simulink model "pid_testing"  (R2019b)
settings: Solver=VariableStepAuto  StartTime=0.0  StopTime=200  RelTol=1e-3
values from neighbouring files (symbols this model uses):
  B_s = 1.0e5    (= 100000)    [PID.m]
  FF_Pitch_Table = [0, 3.5, 6.0, 8.2, 10.4, 12.3, 14.0, 15.5, 18.2, 20.5, 22.5, 23.5]    [setup_model.m]
  FF_Wind_Axis = [11, 12, 13, 14, 15, 16, 17, 18, 20, 22, 24, 25]    [setup_model.m]
  J_g = 3.0e4    (= 30000)    [PID.m]
  J_r = 4.0e6    (= 4000000)    [PID.m]
  K_s = 2.0e6    (= 2000000)    [PID.m]
  Ki = (omega_n)^2 * J_r    (= 1000000)    [PID.m]
  Kp = 2 * zeta * omega_n * J_r    (= 2800000)    [PID.m]
  omega_rated = 2.0    (= 2)    [PID.m]
  R = 40    [PID.m]    (also in gen_dataset_from_sim.m)
  rho = 1.225    [PID.m]
  T_gen_max = 8.0e5    (= 800000)    [PID.m]
  T_gen_min = 0    [PID.m]
  T_gen_rated = 5.0e5    (= 500000)    [PID.m]
  tau_act = 0.05    [PID.m]
  tau_ff = 2.0    (= 2)    [setup_model.m]
libraries: simulink x4, eeGeneralControl x1
settings Model: Creator=Admin  LastModifiedBy=Admin
settings SolverCC: ZeroCrossAlgorithm=Adaptive
settings DebuggingCC: IgnoredZcDiagnostic=none

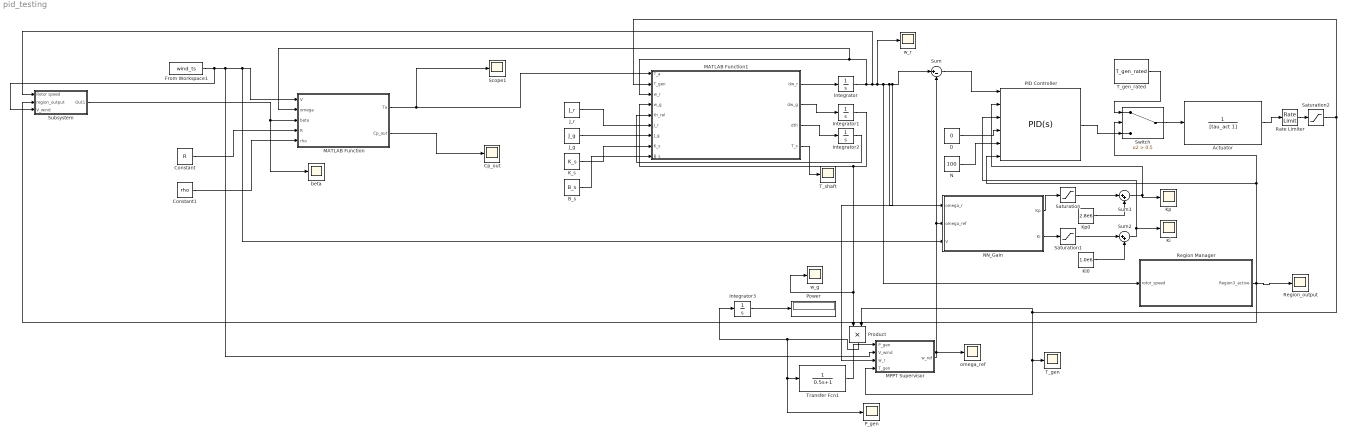
== system pid_testing ==
  Actuator : TransferFcn  Denominator=[tau_act 1]
  B_s : Constant  Value=B_s
  Constant : Constant  Value=R
  Constant1 : Constant  Value=rho
  "Cp_out " : Scope
  D : Constant  Value=0
  From Workspace1 : FromWorkspace  VariableName=wind_ts  SampleTime=0.001
  Integrator : Integrator  InitialCondition=1.5
  Integrator1 : Integrator
  Integrator2 : Integrator
  Integrator3 : Integrator
  J_g : Constant  Value=J_g
  J_r : Constant  Value=J_r
  K_s : Constant  Value=K_s
  "Ki " : Scope
  Ki0 : Constant  Value=1.0e6
  Kp : Scope
  Kp0 : Constant  Value=2.8e6
  MATLAB Function : MATLAB Function  TreatAsAtomicUnit=on
  MATLAB Function1 : MATLAB Function  TreatAsAtomicUnit=on
  "MPPT Supervisor " : Subsystem
  "N " : Constant  Value=100
  "NN_Gain " : MATLAB Function  TreatAsAtomicUnit=on
  PID Controller : simulink/Continuous/PID Controller  Controller=PID  Form=Parallel  TimeDomain=Continuous-time  SampleTime=-1  IntegratorMethod=Forward Euler  FilterMethod=Forward Euler  ControllerParametersSource=external  P=Kp  I=Ki  D=0  UseFilter=on  N=100  TunerSelectOption=Transfer Function Based (PID Tuner App)  InitialConditionSource=internal  InitialConditionForIntegrator=0  InitialConditionForFilter=0  DifferentiatorICPrevScaledInput=0  ExternalReset=level  TrackingMode=off  Kt=1  LimitOutput=on  UpperSaturationLimit=T_gen_max  LowerSaturationLimit=T_gen_min  LinearizeAsGain=on  AntiWindupMode=back-calculation  Kb=0.2  POutMin=[]  POutMax=[]  IOutMin=[]  IOutMax=[]  DOutMin=[]  DOutMax=[]  NOutMin=[]  NOutMax=[]  SumOutMin=[]  SumOutMax=[]  SaturationOutMin=[]  SaturationOutMax=[]  PParamMin=[]  PParamMax=[]  IParamMin=[]  IParamMax=[]  DParamMin=[]  DParamMax=[]  NParamMin=[]  NParamMax=[]  KbParamMin=[]  KbParamMax=[]  KtParamMin=[]  KtParamMax=[]  KbOutMin=[]  KbOutMax=[]  KtOutMin=[]  KtOutMax=[]  IntegratorOutMin=[]  IntegratorOutMax=[]  FilterOutMin=[]  FilterOutMax=[]  SumI1OutMin=[]  SumI1OutMax=[]  SumI2OutMin=[]  SumI2OutMax=[]  SumI3OutMin=[]  SumI3OutMax=[]  SumI4OutMin=[]  SumI4OutMax=[]  SumDOutMin=[]  SumDOutMax=[]  DifferentiatorOutMin=[]  DifferentiatorOutMax=[]  FilterDiffOutCoefMin=[]  FilterDiffOutCoefMax=[]  ReciprocalOutMin=[]  ReciprocalOutMax=[]  SumDenOutMin=[]  SumDenOutMax=[]  SumNumOutMin=[]  SumNumOutMax=[]  DivideOutMin=[]  DivideOutMax=[]  IntegratorContinuousStateAttributes=''  IntegratorStateMustResolveToSignalObject=off  IntegratorRTWStateStorageClass=Auto  FilterContinuousStateAttributes=''  FilterStateMustResolveToSignalObject=off  FilterRTWStateStorageClass=Auto  ParallelPVariant=ExternalParameters  IdealPVariant=Disabled  IVariant=ExternalParameters  DVariant=ExternalParameters  IntegratorVariant=Continuous  SatVariant=Enabled  AWVariant=BackCalculation  PCopyVariant=Disabled  TRVariant=Disabled  FdbkBlocksVariant=Forward  IdealPFdbkVariant=Disabled  SatFdbkVariant=Disabled  DerivativeFilterVariant=ContFilter  NVariant=ExternalParameters  NCopyVariant=Disabled  FilterICVariant=InternalICsFilter  IntegratorICVariant=InternalICs  ExternalResetVariant=ExternalReset  TRSumVariant=Passthrough  SumFdbkVariant=Disabled  SumVariant=Sum_PID
  "P_gen " : Scope
  Power : Display
  Product : Product
  Rate Limiter : RateLimiter  RisingSlewLimit=1e5  FallingSlewLimit=-1e5  SampleTimeMode=inherited
  Region Manager : Subsystem
  "Region_output " : Scope
  Saturation : Saturate  UpperLimit=8.4e5  LowerLimit=-8.4e5
  Saturation1 : Saturate  UpperLimit=3e5  LowerLimit=-3e5
  Saturation2 : Saturate  UpperLimit=8e5  LowerLimit=-8e5
  Scope1 : Scope
  Subsystem : Subsystem
  Sum : Sum  Inputs=|+-
  Sum1 : Sum  Inputs=|++
  Sum2 : Sum  Inputs=|++
  Switch : Switch  Criteria=u2 > Threshold  Threshold=0.5
  "T_gen " : Scope
  "T_gen_rated " : Constant  Value=T_gen_rated
  T_shaft : Scope
  Transfer Fcn1 : TransferFcn  Denominator=[0.5 1]
  beta : Scope
  omega_ref : Scope
  w_g : Scope
  w_r : Scope
  wires:
  MATLAB Function/1(Ta) -> Scope1/1, MATLAB Function1/1(T_a)
  Constant/1 -> MATLAB Function/4(R)
  Constant1/1 -> MATLAB Function/5(rho)
  MATLAB Function/2(Cp_out) -> "Cp_out "/1
  MATLAB Function1/3(dth) -> Integrator2/1
  MATLAB Function1/2(dw_g) -> Integrator1/1
  MATLAB Function1/1(dw_r) -> Integrator/1
  Integrator1/1 -> MATLAB Function1/4(w_g), w_g/1, Product/1
  Integrator2/1 -> MATLAB Function1/5(th_rel)
  J_r/1 -> MATLAB Function1/6(J_r)
  J_g/1 -> MATLAB Function1/7(J_g)
  K_s/1 -> MATLAB Function1/8(K_s)
  B_s/1 -> MATLAB Function1/9(B_s)
  PID Controller/1 -> Switch/3
  Sum/1 -> PID Controller/1
  D/1 -> PID Controller/4
  "N "/1 -> PID Controller/5
  "NN_Gain "/1(Kp) -> Saturation/1
  "NN_Gain "/2(Ki) -> Saturation1/1
  Saturation/1 -> Sum1/1
  Saturation1/1 -> Sum2/1
  Kp0/1 -> Sum1/2
  Ki0/1 -> Sum2/2
  Sum1/1 -> PID Controller/2, Kp/1
  Sum2/1 -> "Ki "/1, PID Controller/3
  "MPPT Supervisor "/1(w_ref) -> omega_ref/1, Sum/2, "NN_Gain "/2(omega_ref)
  Saturation2/1 -> MATLAB Function1/2(T_gen), "MPPT Supervisor "/4("T_gen "), "T_gen "/1, Product/2
  Product/1 -> "P_gen "/1, Transfer Fcn1/1, Integrator3/1
  Transfer Fcn1/1 -> "MPPT Supervisor "/1("P_gen ")
  Actuator/1 -> Rate Limiter/1
  From Workspace1/1 -> Subsystem/3("V_wind "), "MPPT Supervisor "/2("V_wind "), "NN_Gain "/3(V), MATLAB Function/1(V)
  "T_gen_rated "/1 -> Switch/1
  Switch/1 -> Actuator/1
  Subsystem/1(Out1) -> MATLAB Function/3(beta), beta/1
  Integrator3/1 -> Power/1
  Rate Limiter/1 -> Saturation2/1
  MATLAB Function1/4(T_s) -> T_shaft/1
  Region Manager/1("Region3_active ") -> Subsystem/2(region_output), "Region_output "/1, PID Controller/6, Switch/2
  Integrator/1 -> Subsystem/1(Rotor speed), Region Manager/1("rotor_speed "), "MPPT Supervisor "/3(w_r), Sum/1, "NN_Gain "/1(omega_r), w_r/1, MATLAB Function/2(omega), MATLAB Function1/3(w_r)

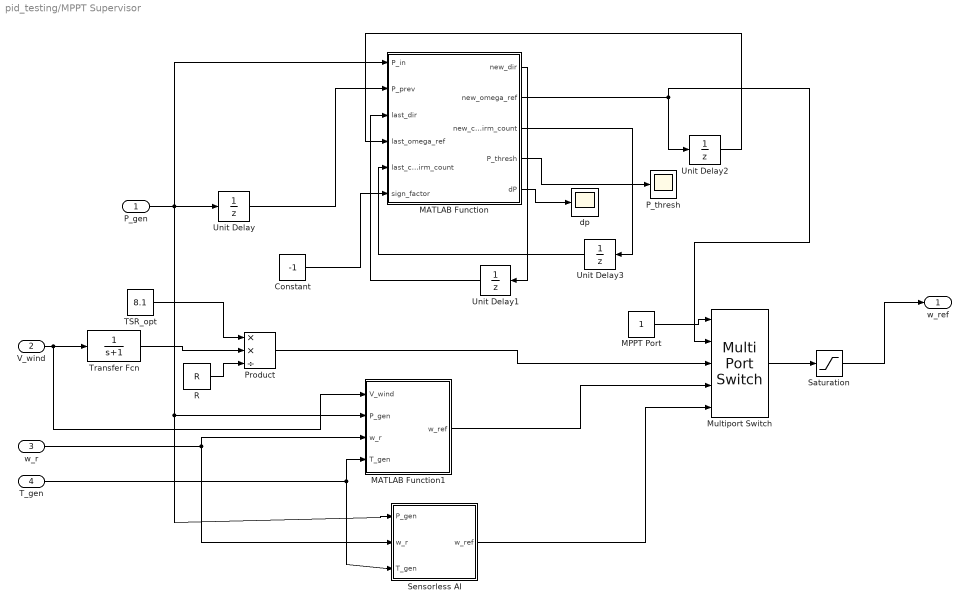
== system pid_testing/MPPT Supervisor  ==
  "P_gen " : Inport
  "V_wind " : Inport  Port=2
  w_r : Inport  Port=3
  "T_gen " : Inport  Port=4
  Constant : Constant  Value=-1
  MATLAB Function : MATLAB Function  TreatAsAtomicUnit=on
  MATLAB Function1 : MATLAB Function  TreatAsAtomicUnit=on
  MPPT Port : Constant
  Multiport Switch : MultiPortSwitch  Inputs=4
  P_thresh : Scope
  Product : Product  Inputs=**/
  "R " : Constant  Value=R
  Saturation : Saturate  UpperLimit=2.2  LowerLimit=0.7
  "Sensorless AI " : MATLAB Function  TreatAsAtomicUnit=on
  "TSR_opt " : Constant  Value=8.1
  Transfer Fcn : TransferFcn  Denominator=[1 1]
  Unit Delay : UnitDelay  HasFrameUpgradeWarning=on
  Unit Delay1 : UnitDelay  InitialCondition=1  HasFrameUpgradeWarning=on
  Unit Delay2 : UnitDelay  InitialCondition=1.5  HasFrameUpgradeWarning=on
  Unit Delay3 : UnitDelay  HasFrameUpgradeWarning=on
  "dp " : Scope
  w_ref : Outport
  wires:
  "P_gen "/1 -> "Sensorless AI "/1(P_gen), MATLAB Function1/2(P_gen), MATLAB Function/1(P_in), Unit Delay/1
  MATLAB Function/1(new_dir) -> Unit Delay1/1
  Unit Delay/1 -> MATLAB Function/2(P_prev)
  Unit Delay1/1 -> MATLAB Function/3(last_dir)
  Unit Delay2/1 -> MATLAB Function/4(last_omega_ref)
  Unit Delay3/1 -> MATLAB Function/5(last_confirm_count)
  Constant/1 -> MATLAB Function/6(sign_factor)
  MATLAB Function/2(new_omega_ref) -> Multiport Switch/2, Unit Delay2/1
  MATLAB Function/3(new_confirm_count) -> Unit Delay3/1
  MATLAB Function/4(P_thresh) -> P_thresh/1
  MATLAB Function/5(dP) -> "dp "/1
  "R "/1 -> Product/3
  "V_wind "/1 -> MATLAB Function1/1(V_wind), Transfer Fcn/1
  "TSR_opt "/1 -> Product/1
  Transfer Fcn/1 -> Product/2
  Product/1 -> Multiport Switch/3
  Multiport Switch/1 -> Saturation/1
  MPPT Port/1 -> Multiport Switch/1
  Saturation/1 -> w_ref/1
  w_r/1 -> MATLAB Function1/3(w_r), "Sensorless AI "/2(w_r)
  "T_gen "/1 -> MATLAB Function1/4(T_gen), "Sensorless AI "/3(T_gen)
  MATLAB Function1/1(w_ref) -> Multiport Switch/4
  "Sensorless AI "/1(w_ref) -> Multiport Switch/5

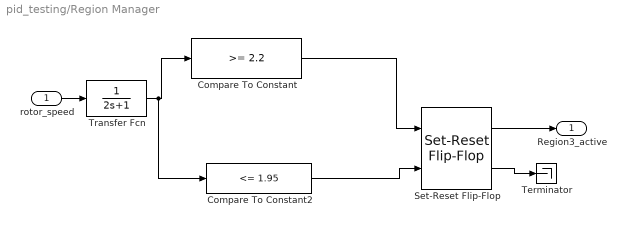
== system pid_testing/Region Manager ==
  "rotor_speed " : Inport
  Compare To Constant : simulink/Logic and Bit Operations/Compare To Constant  relop=>=  const=2.2  OutDataTypeStr=boolean
  Compare To Constant2 : simulink/Logic and Bit Operations/Compare To Constant  relop=<=  const=1.95  OutDataTypeStr=boolean
  Set-Reset Flip-Flop : eeGeneralControl/Set-Reset Flip-Flop  LabelModeActiveChoice=Discrete  UndefState=Set  Q0=0  Ts=-1
      settings: SourceProductName=Simscape Electrical  SourceProductBaseCode=PS
  Terminator : Terminator
  Transfer Fcn : TransferFcn  Denominator=[2 1]
  "Region3_active " : Outport
  wires:
  "rotor_speed "/1 -> Transfer Fcn/1
  Compare To Constant/1 -> Set-Reset Flip-Flop/1
  Compare To Constant2/1 -> Set-Reset Flip-Flop/2
  Set-Reset Flip-Flop/1 -> "Region3_active "/1
  Set-Reset Flip-Flop/2 -> Terminator/1
  Transfer Fcn/1 -> Compare To Constant2/1, Compare To Constant/1

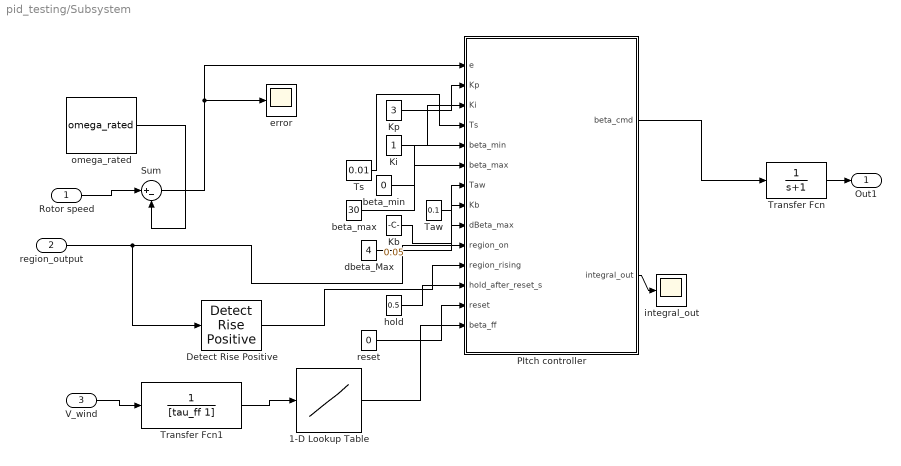
== system pid_testing/Subsystem ==
  Rotor speed : Inport
  region_output : Inport  Port=2
  "V_wind " : Inport  Port=3
  1-D Lookup Table : Lookup_n-D  NumberOfTableDimensions=1  BreakpointsForDimension1=FF_Wind_Axis  Table=FF_Pitch_Table  InternalRulePriority=Speed  RndMeth=Simplest  InputSameDT=on
  Detect Rise Positive : simulink/Logic and Bit Operations/Detect Rise Positive  vinit=0  OutDataTypeStr=boolean
  Kb : Constant  Value=0.05
  Ki : Constant
  Kp : Constant  Value=3
  "PItch controller " : MATLAB Function  TreatAsAtomicUnit=on
  Sum : Sum  Inputs=|+-
  Taw : Constant  Value=0.1
  Transfer Fcn : TransferFcn  Denominator=[1 1]
  Transfer Fcn1 : TransferFcn  Denominator=[tau_ff 1]
  Ts : Constant  Value=0.01
  beta_max : Constant  Value=30
  beta_min : Constant  Value=0
  dbeta_Max : Constant  Value=4
  error : Scope
  hold : Constant  Value=0.5
  "integral_out " : Scope
  "omega_rated " : Constant  Value=omega_rated
  reset : Constant  Value=0
  Out1 : Outport
  wires:
  Rotor speed/1 -> Sum/1
  "omega_rated "/1 -> Sum/2
  Transfer Fcn/1 -> Out1/1
  Sum/1 -> error/1, "PItch controller "/1(e)
  region_output/1 -> Detect Rise Positive/1, "PItch controller "/10(region_on)
  Kp/1 -> "PItch controller "/2(Kp)
  Ki/1 -> "PItch controller "/3(Ki)
  Ts/1 -> "PItch controller "/4(Ts)
  beta_min/1 -> "PItch controller "/5(beta_min)
  beta_max/1 -> "PItch controller "/6(beta_max)
  Taw/1 -> "PItch controller "/7(Taw)
  Kb/1 -> "PItch controller "/8(Kb)
  dbeta_Max/1 -> "PItch controller "/9(dBeta_max)
  hold/1 -> "PItch controller "/12(hold_after_reset_s)
  reset/1 -> "PItch controller "/13(reset)
  "PItch controller "/1(beta_cmd) -> Transfer Fcn/1
  "PItch controller "/2(integral_out) -> "integral_out "/1
  Detect Rise Positive/1 -> "PItch controller "/11(region_rising)
  "V_wind "/1 -> Transfer Fcn1/1
  Transfer Fcn1/1 -> 1-D Lookup Table/1
  1-D Lookup Table/1 -> "PItch controller "/14(beta_ff)

== matlab function pid_testing/MATLAB Function1 ==
  data: T_a input; dw_r output; dw_g output; dth output; T_gen input; w_r input; w_g input; th_rel input; J_r input; J_g input; K_s input; B_s input; T_s output
function [dw_r, dw_g, dth,T_s] = two_mass_dynamics_derivatives(T_a, T_gen, w_r, w_g, th_rel, J_r, J_g, K_s, B_s)
    % This function now calculates DERIVATIVES, not states.

    % Parameters (can be passed in or defined here)


    % Shaft torque calculation (based on current states)
    T_s = K_s * th_rel + B_s * (w_r - w_g);

    % Output the derivatives
    dw_r = (T_a - T_s) / J_r;
    dw_g = (T_s - T_gen) / J_g;
    dth  = w_r - w_g;
end

== matlab function pid_testing/MATLAB Function ==
  data: V input; Ta output; omega input; beta input; R input; Cp_out output; rho input
function [Ta, Cp_out] = aero_torque(V, omega, beta, R, rho)
%#codegen
% Aero torque using analytic Cp; no structs/buses required.
% Inputs:
%   V     - wind speed [m/s]
%   omega - rotor speed [rad/s]
%   beta  - pitch [deg]
%   R     - rotor radius [m]
%   rho   - air density [kg/m^3]
% Outputs:
%   Ta    - aerodynamic torque [N*m]
%   Cp_out- power coefficient (dimensionless)

% Protect inputs
if V <= 1e-6
    V = 1e-6;
end
if omega <= 1e-6
    omega = 1e-6;
end
if R <= 0
    R = 40; % fallback
end
if rho <= 0
    rho = 1.225;
end

% Tip-speed ratio
lambda = omega .* R ./ V;

% Analytic Cp coefficients (replace later with your own if needed)
c1 = 0.5176; c2 = 116; c3 = 0.4; c4 = 5; c5 = 21; c6 = 0;
% Compute lambda_i safely (avoid divide by zero)
den = 1./(lambda + 0.08.*beta) - 0.035./(beta.^3 + 1);
den(den==0) = eps;
lambda_i = 1 ./ den;

Cp_out = c1 .* ((c2 ./ lambda_i - c3 .* beta - c4) .* exp(-c5 ./ lambda_i)) + c6 .* lambda;
% enforce physical bounds
Cp_out = max(0, min(Cp_out, 0.59));

% Rotor swept area
A = pi .* R.^2;

% Aerodynamic torque (use omega-safe)
Ta = 0.5 .* rho .* A .* V.^3 .* Cp_out ./ omega;

% If V is essentially zero, set torque to zero
Ta(V < 1e-6) = 0;
end

== matlab function pid_testing/NN_Gain  ==
  settings: updateMethod=DISCRETE  sampleTime=0.1
  data: omega_r input; Kp output; omega_ref input; V input; Ki output
function [Kp, Ki] = NN_GainScheduler(omega_r, omega_ref, V)
%#codegen
% This block calls an external helper function to run the network.

% Tell the Coder that 'runMyNet' is an external MATLAB function
coder.extrinsic('runMyNet');

% --- Pre-allocate all variables for the Coder ---
% This prevents any "undefined variable" errors.
Kp = 0.0;
Ki = 0.0;
K  = zeros(2,1); % K is a 2x1 vector of doubles

% --- Format the inputs ---
x = [omega_r; omega_ref; V];

% --- Call the helper function ---
% This passes the inputs to 'runMyNet' and gets the 2x1 'K' vector back.
% All complex network logic is hidden from the Coder.
K = runMyNet(x);

% --- Assign the outputs ---
Kp = K(1);
Ki = K(2);

== matlab function pid_testing/MPPT Supervisor /MATLAB Function ==
  data: P_in input; new_dir output; P_prev input; last_dir input; last_omega_ref input; last_confirm_count input; sign_factor input; new_omega_ref output; new_confirm_count output; P_thresh output; dP output
function [new_dir, new_omega_ref, new_confirm_count, P_thresh, dP] = po_fcn( ...
    P_in, P_prev, last_dir, last_omega_ref, last_confirm_count, sign_factor)
% P&O robust step decision
% Inputs:
%  P_in   - filtered power at current step
%  P_prev - filtered power at previous step (UnitDelay)
%  last_dir - previous perturbation direction (+1 or -1) (UnitDelay)
%  last_omega_ref - previous omega_ref (UnitDelay)
%  last_confirm_count - previous consecutive-sign count (UnitDelay)
%  sign_factor - +1 or -1 to flip ΔP interpretation quickly (tune)
%
% Outputs:
%  new_dir - new perturbation direction (+1 or -1)
%  new_omega_ref - updated omega_ref (already saturated here)
%  new_confirm_count - updated confirmation counter
%  P_thresh - computed deadband threshold
%  dP - change in power (for debug/plot)

%% Parameters (tune these)
base_step = 0.02;        % rad/s base step size
min_step  = 0.01;        % minimum step size
omega_min = 0.7;         % lower bound for omega_ref
omega_max = 2.2;         % upper bound for omega_ref
P_thresh_abs = 100;      % absolute deadband [W]
P_rel_factor = 0.002;    % relative deadband fraction of P_in
confirm_needed = 2;      % require this many consecutive opposite samples to flip

%% Protect inputs
if ~isfinite(P_in), P_in = 0; end
if ~isfinite(P_prev), P_prev = 0; end

%% Compute dP and threshold
dP = P_in - P_prev;
P_thresh = max(P_thresh_abs, P_rel_factor * abs(P_in));

%% Effective dP after applying sign_factor (useful to invert quickly)
dP_eff = sign_factor * dP;

%% Decision logic with deadband and confirmation
% Default keep same direction
new_dir = last_dir;
new_confirm_count = 0;

if abs(dP_eff) < P_thresh
    % within deadband -> do nothing, reset confirm counter
    new_dir = last_dir;
    new_confirm_count = 0;
else
    if dP_eff > 0
        % effective dP positive -> the last step direction was correct
        new_dir = last_dir;
        new_confirm_count = 0;
    else
        % effective dP negative -> candidate to flip
        % require consecutive confirmations to avoid noise flips
        if last_confirm_count + 1 >= confirm_needed
            new_dir = -last_dir;   % flip
            new_confirm_count = 0; % reset after flip
        else
            new_dir = last_dir;    % hold and increment counter
            new_confirm_count = last_confirm_count + 1;
        end
    end
end

%% Compute step (could be adaptive; keep simple stable step)
step = max(min_step, base_step);

%% Update omega_ref using the direction that will be applied *next step*
% (we update based on new_dir so the change is consistent with decision)
new_omega_ref = last_omega_ref + new_dir * step;

% Saturate omega_ref (safety)
if new_omega_ref < omega_min
    new_omega_ref = omega_min;
end
if new_omega_ref > omega_max
    new_omega_ref = omega_max;
end

end

== matlab function pid_testing/Subsystem/PItch controller  ==
  settings: updateMethod=DISCRETE  sampleTime=0.01
  data: e input; beta_cmd output; Kp input; Ki input; Ts input; beta_min input; beta_max input; Taw input; Kb input; dBeta_max input; region_on input; region_rising input; hold_after_reset_s input; integral_out output; reset input; beta_ff input
function [beta_cmd, integral_out] = pitch_PI_safe(e, Kp, Ki, Ts, ...
    beta_min, beta_max, Taw, Kb, dBeta_max, region_on, region_rising, hold_after_reset_s, reset, beta_ff)
% Safe PI: anti-windup, conditional integrate, soft reset/unwind while held
% (Units: beta in degrees or same units used in model)
if ~region_on
    beta_ff = 0;
end

% ---- DEFAULT PARAMS (tune as needed) ----
if nargin < 13
    hold_after_reset_s = 0.5;
end
% -----------------------------------------

persistent integral prev_beta hold_counter
if isempty(integral)
    integral = 0; prev_beta = 0; hold_counter = 0;
end
if reset
    integral = 0; prev_beta = 0; hold_counter = 0;
end

% on rising edge: soft reset (set integral to value that avoids command jump)
if region_rising
    % Option A: hard reset
    % integral = 0;
    % Option B (soft preload) - set integral so u_total equals current actuator pos (preload)
    % assume we have access to current beta_act (not shown). If not available, fallback to small reset:
    integral = 0;  % start with zero; hold prevents immediate re-wind
    hold_counter = round(hold_after_reset_s / Ts);
end

% decrement hold counter
if hold_counter > 0
    hold_counter = hold_counter - 1;
end
hold_integration = (hold_counter > 0);

% compute P and current unsat output
u_p = Kp * e;
u_pid_unsat = u_p + integral; % PID contribution only

% Total unsaturated command (PID + Feed-Forward)
u_total_unsat = u_pid_unsat + beta_ff;


% saturation (for anti-windup calculation)
u_total_sat = min(max(u_total_unsat, beta_min), beta_max);

u_pid_effective = u_total_sat - beta_ff;

% decide integration allowance
allow_integrate = region_on && (~hold_integration);

% integrator update
if allow_integrate
    % integrate normally
    integral = integral + Ki * Ts * e;
    % back-calculation anti-windup (unwind if saturated)
    if Taw > 0
        % Compare u_pid_effective (what we got) vs u_pid_unsat (what we wanted)
        integral = integral + (Kb * (u_pid_effective - u_pid_unsat)) * (Ts / Taw);
    end
else
    % NOT allowed to integrate: do small unwind toward u_sat rather than hard clamp
    if Taw > 0
        integral = integral + (Kb * (u_pid_effective - u_pid_unsat)) * (Ts / Taw);
    end
end

% clamp integrator to safe bounds (in command units)
Imin = beta_min* -0.6;
Imax = beta_max * 0.6;
integral = min(max(integral, Imin), Imax);

% compute total command and rate-limit
% Rate limit the TOTAL saturated command
% We use u_total_sat as the target
max_delta = dBeta_max * Ts;
delta = u_total_sat - prev_beta;

if delta > max_delta
    beta_final = prev_beta + max_delta;
elseif delta < -max_delta
    beta_final = prev_beta - max_delta;
else
    beta_final = u_total_sat;
end

% Final safety saturation (redundant but good practice)
beta_cmd = min(max(beta_final, beta_min), beta_max);

prev_beta = beta_cmd;
integral_out = integral;
end

== matlab function pid_testing/MPPT Supervisor /MATLAB Function1 ==
  settings: updateMethod=DISCRETE  sampleTime=0.1
  data: V_wind input; w_ref output; P_gen input; w_r input; T_gen input
function w_ref = AI_MPPT(V_wind, P_gen, w_r, T_gen)
%#codegen

% Tell Simulink that run_AE_MPPT is an external MATLAB file
coder.extrinsic('run_AE_MPPT');

% Prepare the input vector
inputs = [V_wind; P_gen; w_r; T_gen];

% Initialize output for Coder safety
w_ref = 0.0;

% Call the helper function
w_ref = run_AE_MPPT(inputs);

== matlab function pid_testing/MPPT Supervisor /Sensorless AI  ==
  settings: updateMethod=DISCRETE  sampleTime=0.1
  data: P_gen input; w_ref output; w_r input; T_gen input
function w_ref = Sensorless_AI(P_gen, w_r, T_gen)
%#codegen

% Tell Simulink to use the external helper file
coder.extrinsic('run_sensorless_AI');

% Prepare input vector
inputs = [P_gen; w_r; T_gen];

% Initialize output for Coder safety
w_ref = 0.0;

% Call the brain
w_ref = run_sensorless_AI(inputs);

end
